simulink model "Week1Problem5"  (R2020b)
settings: Solver=VariableStepAuto  StartTime=0.0  StopTime=10.0  RelTol=1e-3
values from neighbouring files (symbols this model uses):
  R = 10    [rcvalue.m]
undefined symbols (not defined in the file or in its folder): C
settings Model: Creator=HP  LastModifiedBy=HP

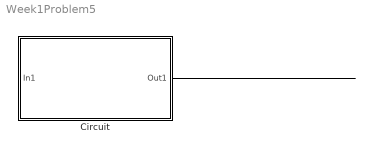
== system Week1Problem5 ==
  Circuit : Subsystem
  wires:
  ? -> Circuit/1(In1)  "E(t)"
  Circuit/1(Out1) -> ?

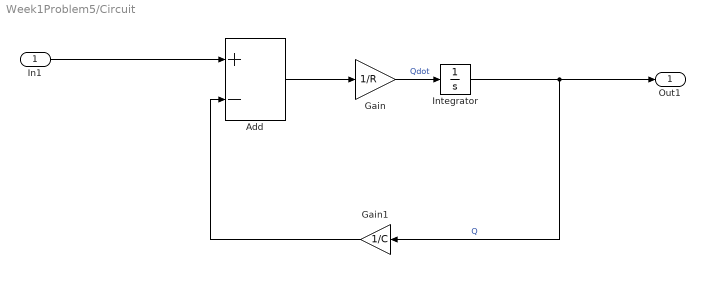
== system Week1Problem5/Circuit ==
  In1 : Inport
  Add : Sum  Inputs=+-
  Gain : Gain  Gain=1/R
  Gain1 : Gain  Gain=1/C
  Integrator : Integrator  InitialCondition=500
  Out1 : Outport
  wires:
  Gain1/1 -> Add/2
  Gain/1 -> Integrator/1  "Qdot"
  In1/1 -> Add/1
  Add/1 -> Gain/1
  Integrator/1 -> Out1/1, Gain1/1  "Q"
